simulink model "Filter"  (Simulink 6.5)
settings: Solver=FixedStepDiscrete  StartTime=0.0  StopTime=10.0  RelTol=1e-3
undefined symbols (not defined in the file): dfilt
libraries: dsparch4 x71
(part 1 of 3)
settings Model: Creator=cameraman  LastModifiedBy=cameraman  ExtModeAutoUpdateStatusClock=off
settings OptimizationCC: OptimizeModelRefInitCode=on  LifeSpan=1
settings RTWCC: SystemTargetFile=ert.tlc  TemplateMakefile=ert_default_tmf  Description=Real-Time Workshop Embedded Coder (no auto configuration)  GenerateReport=on  ProcessScript=ert_make_rtw_hook  IncludeHyperlinkInReport=on  LaunchReport=on
settings CodeAppCC: IgnoreCustomStorageClasses=off
settings ERTTargetCC: TargetFcnLib=ansi_tfl_tmw.mat  GenFloatMathFcnCalls=ANSI_C  GenerateSampleERTMain=on  InlinedParameterPlacement=NonHierarchical  ERTCustomFileTemplate=example_file_process.tlc

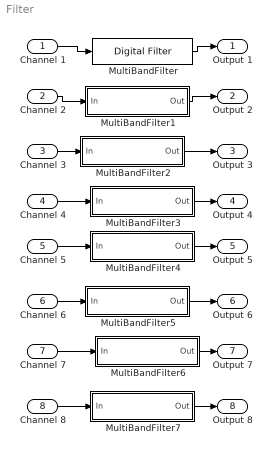
== system Filter ==
  Channel 1 : Inport  PortDimensions=[400 1]  DataType=single
  Channel 2 : Inport  Port=2  PortDimensions=[400 1]  DataType=single
  Channel 3 : Inport  Port=3  PortDimensions=[400 1]  DataType=single
  Channel 4 : Inport  Port=4  PortDimensions=[400 1]  DataType=single
  Channel 5 : Inport  Port=5  PortDimensions=[400 1]  DataType=single
  Channel 6 : Inport  Port=6  PortDimensions=[400 1]  DataType=single
  Channel 7 : Inport  Port=7  PortDimensions=[400 1]  DataType=single
  Channel 8 : Inport  Port=8  PortDimensions=[400 1]  DataType=single
  MultiBandFilter : dsparch4/Digital Filter  Tag=BlockMethodSubSystem  DialogController=dspdialog.DigitalFilter  DialogControllerArgs=DataTag0  TypePopup=IIR (poles & zeros)  IIRFiltStruct=Biquad direct form II (SOS)  AllPoleFiltStruct=Direct form  FIRFiltStruct=Direct form  CoeffSource=Specify via dialog  NumCoeffs=[1 2]  DenCoeffs=[1 0.1]  BiQuadCoeffs=[1 -1.99751859287897 1 1 -1.99114673192373 0.993753760540243;1 -1.99804090685014 0.999999999999999 1 -1.99287686475877 0.994730821052702]  LatticeCoeffs=[0.2 0.4]  denIgnore=on  FiltPerSampPopup=One filter per frame  IC=0  ICnum=0  ICden=0  roundingMode=Floor  overflowMode=off  ScaleValues=[0.994242170508505;1;1]  scaleValueFracLength=14  stageInFracLength=15  stageOutFracLength=15  FilterSource=Specify via dialog  dfiltObjectName=dfilt.dffir([1 2 1])
  MultiBandFilter1 : Subsystem  Tag=BlockMethodSubSystem
  MultiBandFilter2 : Subsystem  Tag=BlockMethodSubSystem
  MultiBandFilter3 : Subsystem  Tag=BlockMethodSubSystem
  MultiBandFilter4 : Subsystem  Tag=BlockMethodSubSystem
  MultiBandFilter5 : Subsystem  Tag=BlockMethodSubSystem
  MultiBandFilter6 : Subsystem  Tag=BlockMethodSubSystem
  MultiBandFilter7 : Subsystem  Tag=BlockMethodSubSystem
  Output 1 : Outport
  Output 2 : Outport  Port=2
  Output 3 : Outport  Port=3
  Output 4 : Outport  Port=4
  Output 5 : Outport  Port=5
  Output 6 : Outport  Port=6
  Output 7 : Outport  Port=7
  Output 8 : Outport  Port=8
  wires:
  Channel 1/1 -> MultiBandFilter/1
  MultiBandFilter/1 -> Output 1/1
  Channel 2/1 -> MultiBandFilter1/1(In)
  MultiBandFilter1/1(Out) -> Output 2/1
  Channel 3/1 -> MultiBandFilter2/1(In)
  MultiBandFilter2/1(Out) -> Output 3/1
  Channel 4/1 -> MultiBandFilter3/1(In)
  MultiBandFilter3/1(Out) -> Output 4/1
  Channel 5/1 -> MultiBandFilter4/1(In)
  MultiBandFilter4/1(Out) -> Output 5/1
  Channel 6/1 -> MultiBandFilter5/1(In)
  MultiBandFilter5/1(Out) -> Output 6/1
  Channel 7/1 -> MultiBandFilter6/1(In)
  MultiBandFilter6/1(Out) -> Output 7/1
  Channel 8/1 -> MultiBandFilter7/1(In)
  MultiBandFilter7/1(Out) -> Output 8/1

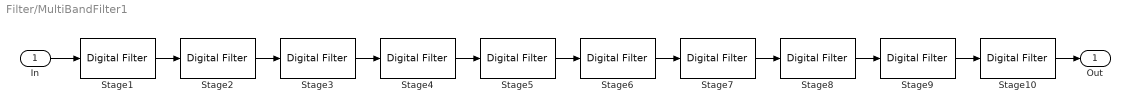
== system Filter/MultiBandFilter1 ==
  In : Inport
  Stage1 : dsparch4/Digital Filter  Tag=BlockMethodSubSystem  DialogController=dspdialog.DigitalFilter  DialogControllerArgs=DataTag1  TypePopup=IIR (poles & zeros)  IIRFiltStruct=Biquad direct form II (SOS)  AllPoleFiltStruct=Direct form  FIRFiltStruct=Direct form  CoeffSource=Specify via dialog  NumCoeffs=[1 2]  DenCoeffs=[1 0.1]  BiQuadCoeffs=[1 -1.99779918117944 1 1 -1.9841893580212 0.986532671822607;1 -1.99779918117944 1 1 -1.9844084470834 0.986594514381433;1 -1.99779918117944 1 1 -1.98482594276861 0.987328003055499;1 -1.99779918117944 1 1 -1.98539047342403 0.987430635535995;1 -1.99779918117944 1 1 -1.98700178992716 0.98891468957857;1 -1.99779918117944 1 1 -1.98634462539793 0.988995338567042;1 -1.99779918117944 1 1 -1.98909486873423 0.990903795973587;1 -1.99779918117944 1 1 -1.98868956515963 0.991466803510252;1 -1.99779918117944 1 1 -1.99152919723188 0.993259885911427;1 -1.99779918117944 1 1 -1.99172030080645 0.994590980134811;1 -1.99779918117944 1 1 -1.99418204154646 0.9958611964492;1 -1.99779918117944 1 1 -1.99522268630609 0.998145251526606;1 -1.99779918117944 1 1 -1.99694953271705 0.998604078200721]  LatticeCoeffs=[0.2 0.4]  denIgnore=on  FiltPerSampPopup=One filter per frame  IC=0  ICnum=0  ICden=0  roundingMode=Floor  overflowMode=off  ScaleValues=[0.94555573617425;1;1;1;1;1;1;1;1;1;1;1;1;1]  scaleValueFracLength=14  stageInFracLength=15  stageOutFracLength=15  FilterSource=Specify via dialog  dfiltObjectName=dfilt.dffir([1 2 1])
  Stage10 : dsparch4/Digital Filter  Tag=BlockMethodSubSystem  DialogController=dspdialog.DigitalFilter  DialogControllerArgs=DataTag2  TypePopup=IIR (poles & zeros)  IIRFiltStruct=Biquad direct form II (SOS)  AllPoleFiltStruct=Direct form  FIRFiltStruct=Direct form  CoeffSource=Specify via dialog  NumCoeffs=[1 2]  DenCoeffs=[1 0.1]  BiQuadCoeffs=[1 -1.78206655900016 1 1 -1.76882371693892 0.986071932968289;1 -1.78206655900016 1 1 -1.77053018639569 0.986121890411467;1 -1.78206655900016 1 1 -1.76800612910907 0.986970023612059;1 -1.78206655900016 1 1 -1.77300273862414 0.987106634145622;1 -1.78206655900016 1 1 -1.76814322166804 0.988766014578574;1 -1.78206655900016 1 1 -1.776071635619 0.98895295803498;1 -1.78206655900016 1 1 -1.7692366984374 0.991346893216688;1 -1.78206655900016 1 1 -1.77953211525407 0.991534308059337;1 -1.78206655900016 1 1 -1.77122117194367 0.994542018120079;1 -1.78206655900016 1 1 -1.78315724552427 0.994679643471267;1 -1.78206655900016 1 1 -1.77396619462103 0.998133320751102;1 -1.78206655900016 1 1 -1.78671109622842 0.998183872576326]  LatticeCoeffs=[0.2 0.4]  denIgnore=on  FiltPerSampPopup=One filter per frame  IC=0  ICnum=0  ICden=0  roundingMode=Floor  overflowMode=off  ScaleValues=[0.947343827190167;1;1;1;1;1;1;1;1;1;1;1;1]  scaleValueFracLength=14  stageInFracLength=15  stageOutFracLength=15  FilterSource=Specify via dialog  dfiltObjectName=dfilt.dffir([1 2 1])
  Stage2 : dsparch4/Digital Filter  Tag=BlockMethodSubSystem  DialogController=dspdialog.DigitalFilter  DialogControllerArgs=DataTag3  TypePopup=IIR (poles & zeros)  IIRFiltStruct=Biquad direct form II (SOS)  AllPoleFiltStruct=Direct form  FIRFiltStruct=Direct form  CoeffSource=Specify via dialog  NumCoeffs=[1 2]  DenCoeffs=[1 0.1]  BiQuadCoeffs=[1 -1.99114895169414 1 1 -1.9777698136482 0.986561389056741;1 -1.99114895169414 1 1 -1.97762596482961 0.986726523617136;1 -1.99114895169414 1 1 -1.97867590148041 0.987172279710376;1 -1.99114895169414 1 1 -1.97829191516836 0.987696909569038;1 -1.99114895169414 1 1 -1.98025580346007 0.98848655327017;1 -1.99114895169414 1 1 -1.97976262159325 0.989447779407759;1 -1.99114895169414 1 1 -1.98239359272873 0.990400910611987;1 -1.99114895169414 1 1 -1.98197315937799 0.99189471261422;1 -1.99114895169414 1 1 -1.98495805169617 0.992793520063566;1 -1.99114895169414 1 1 -1.98479800244236 0.994894776562119;1 -1.99114895169414 1 1 -1.98781178283368 0.995533402367328;1 -1.99114895169414 1 1 -1.98805774118811 0.998255069724644;1 -1.99114895169414 1 1 -1.99081649186752 0.998486141008158]  LatticeCoeffs=[0.2 0.4]  denIgnore=on  FiltPerSampPopup=One filter per frame  IC=0  ICnum=0  ICden=0  roundingMode=Floor  overflowMode=off  ScaleValues=[0.945424059198097;1;1;1;1;1;1;1;1;1;1;1;1;1]  scaleValueFracLength=14  stageInFracLength=15  stageOutFracLength=15  FilterSource=Specify via dialog  dfiltObjectName=dfilt.dffir([1 2 1])
  Stage3 : dsparch4/Digital Filter  Tag=BlockMethodSubSystem  DialogController=dspdialog.DigitalFilter  DialogControllerArgs=DataTag4  TypePopup=IIR (poles & zeros)  IIRFiltStruct=Biquad direct form II (SOS)  AllPoleFiltStruct=Direct form  FIRFiltStruct=Direct form  CoeffSource=Specify via dialog  NumCoeffs=[1 2]  DenCoeffs=[1 0.1]  BiQuadCoeffs=[1 -1.98008133141043 1 1 -1.96672531746014 0.98650963095461;1 -1.98008133141043 1 1 -1.9665032033086 0.986750210536813;1 -1.98008133141043 1 1 -1.96770829457944 0.987048018168876;1 -1.98008133141043 1 1 -1.96708108164623 0.987781888491603;1 -1.98008133141043 1 1 -1.9693722273266 0.988309689218342;1 -1.98008133141043 1 1 -1.96844912868538 0.989566666186125;1 -1.98008133141043 1 1 -1.97160622384232 0.990204155709112;1 -1.98008133141043 1 1 -1.9705438145287 0.992013704878429;1 -1.98008133141043 1 1 -1.97427807467665 0.992615273561397;1 -1.98008133141043 1 1 -1.97324801352515 0.994981712399624;1 -1.98008133141043 1 1 -1.9772425042935 0.995409386053048;1 -1.98008133141043 1 1 -1.97639672748523 0.998286892295906;1 -1.98008133141043 1 1 -1.98034741185451 0.998441686205688]  LatticeCoeffs=[0.2 0.4]  denIgnore=on  FiltPerSampPopup=One filter per frame  IC=0  ICnum=0  ICden=0  roundingMode=Floor  overflowMode=off  ScaleValues=[0.94521834272877;1;1;1;1;1;1;1;1;1;1;1;1;1]  scaleValueFracLength=14  stageInFracLength=15  stageOutFracLength=15  FilterSource=Specify via dialog  dfiltObjectName=dfilt.dffir([1 2 1])
  Stage4 : dsparch4/Digital Filter  Tag=BlockMethodSubSystem  DialogController=dspdialog.DigitalFilter  DialogControllerArgs=DataTag5  TypePopup=IIR (poles & zeros)  IIRFiltStruct=Biquad direct form II (SOS)  AllPoleFiltStruct=Direct form  FIRFiltStruct=Direct form  CoeffSource=Specify via dialog  NumCoeffs=[1 2]  DenCoeffs=[1 0.1]  BiQuadCoeffs=[1 -1.96462073071133 1 1 -1.95131453516727 0.986454183918466;1 -1.96462073071133 1 1 -1.95097599315203 0.986733316047603;1 -1.96462073071133 1 1 -1.95241103954817 0.986957189742735;1 -1.96462073071133 1 1 -1.95143475200162 0.987798186147947;1 -1.96462073071133 1 1 -1.95418555944522 0.988195019819642;1 -1.96462073071133 1 1 -1.95268285779345 0.989604039158267;1 -1.96462073071133 1 1 -1.95652583164486 0.990083454905274;1 -1.96462073071133 1 1 -1.95466134426594 0.992056533195046;1 -1.96462073071133 1 1 -1.95929588143521 0.992509047155787;1 -1.96462073071133 1 1 -1.95726060193215 0.99501482064796;1 -1.96462073071133 1 1 -1.96234396844906 0.995336593760866;1 -1.96462073071133 1 1 -1.96032547879966 0.998299286167002;1 -1.96462073071133 1 1 -1.96550938793341 0.99841576443763]  LatticeCoeffs=[0.2 0.4]  denIgnore=on  FiltPerSampPopup=One filter per frame  IC=0  ICnum=0  ICden=0  roundingMode=Floor  overflowMode=off  ScaleValues=[0.944998002113535;1;1;1;1;1;1;1;1;1;1;1;1;1]  scaleValueFracLength=14  stageInFracLength=15  stageOutFracLength=15  FilterSource=Specify via dialog  dfiltObjectName=dfilt.dffir([1 2 1])
  Stage5 : dsparch4/Digital Filter  Tag=BlockMethodSubSystem  DialogController=dspdialog.DigitalFilter  DialogControllerArgs=DataTag6  TypePopup=IIR (poles & zeros)  IIRFiltStruct=Biquad direct form II (SOS)  AllPoleFiltStruct=Direct form  FIRFiltStruct=Direct form  CoeffSource=Specify via dialog  NumCoeffs=[1 2]  DenCoeffs=[1 0.1]  BiQuadCoeffs=[1 -1.94478249891763 1 1 -1.93168563103253 0.986531277515732;1 -1.94478249891763 1 1 -1.93122059433768 0.98683224264617;1 -1.94478249891763 1 1 -1.93289679174763 0.987008022660797;1 -1.94478249891763 1 1 -1.9315440207779 0.987909159177024;1 -1.94478249891763 1 1 -1.93477174408612 0.988220764886103;1 -1.94478249891763 1 1 -1.93265238090657 0.989713390126836;1 -1.94478249891763 1 1 -1.93719562555007 0.990089878461174;1 -1.94478249891763 1 1 -1.93449307371312 0.99214912798033;1 -1.94478249891763 1 1 -1.94002906949208 0.992504525913789;1 -1.94478249891763 1 1 -1.93696481960067 0.995076908665192;1 -1.94478249891763 1 1 -1.94311601779459 0.995329644404817;1 -1.94478249891763 1 1 -1.93992220998769 0.998321181982756;1 -1.94478249891763 1 1 -1.94629090980952 0.998412672723036]  LatticeCoeffs=[0.2 0.4]  denIgnore=on  FiltPerSampPopup=One filter per frame  IC=0  ICnum=0  ICden=0  roundingMode=Floor  overflowMode=off  ScaleValues=[0.945304374468395;1;1;1;1;1;1;1;1;1;1;1;1;1]  scaleValueFracLength=14  stageInFracLength=15  stageOutFracLength=15  FilterSource=Specify via dialog  dfiltObjectName=dfilt.dffir([1 2 1])
  Stage6 : dsparch4/Digital Filter  Tag=BlockMethodSubSystem  DialogController=dspdialog.DigitalFilter  DialogControllerArgs=DataTag7  TypePopup=IIR (poles & zeros)  IIRFiltStruct=Biquad direct form II (SOS)  AllPoleFiltStruct=Direct form  FIRFiltStruct=Direct form  CoeffSource=Specify via dialog  NumCoeffs=[1 2]  DenCoeffs=[1 0.1]  BiQuadCoeffs=[1 -1.92064508859285 1 1 -1.90765410756011 0.986472273185828;1 -1.92064508859285 1 1 -1.907050442905 0.986789562567385;1 -1.92064508859285 1 1 -1.90899779890478 0.986936076758397;1 -1.92064508859285 1 1 -1.90723446074659 0.987882764412469;1 -1.92064508859285 1 1 -1.91099420923453 0.988142502047033;1 -1.92064508859285 1 1 -1.90820859710794 0.989700395733405;1 -1.92064508859285 1 1 -1.91352351788692 0.990014235945716;1 -1.92064508859285 1 1 -1.90992699967146 0.992144970754847;1 -1.92064508859285 1 1 -1.91644123248104 0.992441250621335;1 -1.92064508859285 1 1 -1.91229576801519 0.995076816055327;1 -1.92064508859285 1 1 -1.91958607166706 0.995287523829068;1 -1.92064508859285 1 1 -1.91517702031526 0.998321590786422;1 -1.92064508859285 1 1 -1.92278752399999 0.998397870496279]  LatticeCoeffs=[0.2 0.4]  denIgnore=on  FiltPerSampPopup=One filter per frame  IC=0  ICnum=0  ICden=0  roundingMode=Floor  overflowMode=off  ScaleValues=[0.94506988263773;1;1;1;1;1;1;1;1;1;1;1;1;1]  scaleValueFracLength=14  stageInFracLength=15  stageOutFracLength=15  FilterSource=Specify via dialog  dfiltObjectName=dfilt.dffir([1 2 1])
  Stage7 : dsparch4/Digital Filter  Tag=BlockMethodSubSystem  DialogController=dspdialog.DigitalFilter  DialogControllerArgs=DataTag8  TypePopup=IIR (poles & zeros)  IIRFiltStruct=Biquad direct form II (SOS)  AllPoleFiltStruct=Direct form  FIRFiltStruct=Direct form  CoeffSource=Specify via dialog  NumCoeffs=[1 2]  DenCoeffs=[1 0.1]  BiQuadCoeffs=[1 -1.89222757165677 1 1 -1.87946492530582 0.986510453032056;1 -1.89222757165677 1 1 -1.87872413047093 0.986838101460465;1 -1.89222757165677 1 1 -1.88093278114135 0.986961705641337;1 -1.89222757165677 1 1 -1.87876382191273 0.987936924736541;1 -1.89222757165677 1 1 -1.88303530627035 0.988156052672692;1 -1.89222757165677 1 1 -1.87959304768991 0.989753596101735;1 -1.89222757165677 1 1 -1.88564809933575 0.990018375641976;1 -1.89222757165677 1 1 -1.88117342448449 0.992189935251698;1 -1.89222757165677 1 1 -1.88862249944903 0.992439907123505;1 -1.89222757165677 1 1 -1.88341916121208 0.995106934972423;1 -1.89222757165677 1 1 -1.89179355317212 0.99528471353657;1 -1.89222757165677 1 1 -1.88620064251826 0.998332207367685;1 -1.89222757165677 1 1 -1.89498786374351 0.998396566697007]  LatticeCoeffs=[0.2 0.4]  denIgnore=on  FiltPerSampPopup=One filter per frame  IC=0  ICnum=0  ICden=0  roundingMode=Floor  overflowMode=off  ScaleValues=[0.945221609871693;1;1;1;1;1;1;1;1;1;1;1;1;1]  scaleValueFracLength=14  stageInFracLength=15  stageOutFracLength=15  FilterSource=Specify via dialog  dfiltObjectName=dfilt.dffir([1 2 1])
  Stage8 : dsparch4/Digital Filter  Tag=BlockMethodSubSystem  DialogController=dspdialog.DigitalFilter  DialogControllerArgs=DataTag9  TypePopup=IIR (poles & zeros)  IIRFiltStruct=Biquad direct form II (SOS)  AllPoleFiltStruct=Direct form  FIRFiltStruct=Direct form  CoeffSource=Specify via dialog  NumCoeffs=[1 2]  DenCoeffs=[1 0.1]  BiQuadCoeffs=[1 -1.85960883542276 1 1 -1.84593411646957 0.986021509148453;1 -1.85960883542276 1 1 -1.84734605082752 0.986086207824345;1 -1.85960883542276 1 1 -1.84544140778377 0.986909714475135;1 -1.85960883542276 1 1 -1.84957097535378 0.987086633043367;1 -1.85960883542276 1 1 -1.84591485590852 0.9887038952601;1 -1.85960883542276 1 1 -1.85245319647007 0.988945992272582;1 -1.85960883542276 1 1 -1.8473354240394 0.991292677324705;1 -1.85960883542276 1 1 -1.85579926237776 0.991535378665241;1 -1.85960883542276 1 1 -1.84961594661188 0.994504963105796;1 -1.85960883542276 1 1 -1.85939042619789 0.994683183912115;1 -1.85960883542276 1 1 -1.85260449337881 0.998120129074157;1 -1.85960883542276 1 1 -1.86299517573272 0.998185591844758]  LatticeCoeffs=[0.2 0.4]  denIgnore=on  FiltPerSampPopup=One filter per frame  IC=0  ICnum=0  ICden=0  roundingMode=Floor  overflowMode=off  ScaleValues=[0.947184039013874;1;1;1;1;1;1;1;1;1;1;1;1]  scaleValueFracLength=14  stageInFracLength=15  stageOutFracLength=15  FilterSource=Specify via dialog  dfiltObjectName=dfilt.dffir([1 2 1])
  Stage9 : dsparch4/Digital Filter  Tag=BlockMethodSubSystem  DialogController=dspdialog.DigitalFilter  DialogControllerArgs=DataTag10  TypePopup=IIR (poles & zeros)  IIRFiltStruct=Biquad direct form II (SOS)  AllPoleFiltStruct=Direct form  FIRFiltStruct=Direct form  CoeffSource=Specify via dialog  NumCoeffs=[1 2]  DenCoeffs=[1 0.1]  BiQuadCoeffs=[1 -1.82286130163383 1 1 -1.8093904390343 0.986049340185928;1 -1.82286130163383 1 1 -1.81095051165661 0.986105875757923;1 -1.82286130163383 1 1 -1.80873514996766 0.986943025633069;1 -1.82286130163383 1 1 -1.81330095324135 0.987097623443224;1 -1.82286130163383 1 1 -1.80904088159003 0.988738220453347;1 -1.82286130163383 1 1 -1.81627907594021 0.988949776437469;1 -1.82286130163383 1 1 -1.81029885913928 0.991322642616634;1 -1.82286130163383 1 1 -1.81968568641089 0.991534729877009;1 -1.82286130163383 1 1 -1.81243274513281 0.994525446348993;1 -1.82286130163383 1 1 -1.82329772701486 0.994681188352925;1 -1.82286130163383 1 1 -1.8153013406224 0.998127421634027;1 -1.82286130163383 1 1 -1.82688113842232 0.998184627861444]  LatticeCoeffs=[0.2 0.4]  denIgnore=on  FiltPerSampPopup=One filter per frame  IC=0  ICnum=0  ICden=0  roundingMode=Floor  overflowMode=off  ScaleValues=[0.947272180688283;1;1;1;1;1;1;1;1;1;1;1;1]  scaleValueFracLength=14  stageInFracLength=15  stageOutFracLength=15  FilterSource=Specify via dialog  dfiltObjectName=dfilt.dffir([1 2 1])
  Out : Outport
  wires:
  In/1 -> Stage1/1
  Stage1/1 -> Stage2/1
  Stage2/1 -> Stage3/1
  Stage3/1 -> Stage4/1
  Stage4/1 -> Stage5/1
  Stage5/1 -> Stage6/1
  Stage6/1 -> Stage7/1
  Stage7/1 -> Stage8/1
  Stage8/1 -> Stage9/1
  Stage9/1 -> Stage10/1
  Stage10/1 -> Out/1

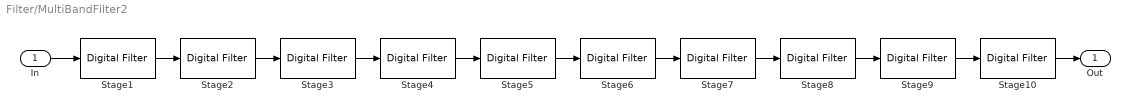
== system Filter/MultiBandFilter2 ==
  In : Inport
  Stage1 : dsparch4/Digital Filter  Tag=BlockMethodSubSystem  DialogController=dspdialog.DigitalFilter  DialogControllerArgs=DataTag11  TypePopup=IIR (poles & zeros)  IIRFiltStruct=Biquad direct form II (SOS)  AllPoleFiltStruct=Direct form  FIRFiltStruct=Direct form  CoeffSource=Specify via dialog  NumCoeffs=[1 2]  DenCoeffs=[1 0.1]  BiQuadCoeffs=[1 -1.99779918117944 1 1 -1.9841893580212 0.986532671822607;1 -1.99779918117944 1 1 -1.9844084470834 0.986594514381433;1 -1.99779918117944 1 1 -1.98482594276861 0.987328003055499;1 -1.99779918117944 1 1 -1.98539047342403 0.987430635535995;1 -1.99779918117944 1 1 -1.98700178992716 0.98891468957857;1 -1.99779918117944 1 1 -1.98634462539793 0.988995338567042;1 -1.99779918117944 1 1 -1.98909486873423 0.990903795973587;1 -1.99779918117944 1 1 -1.98868956515963 0.991466803510252;1 -1.99779918117944 1 1 -1.99152919723188 0.993259885911427;1 -1.99779918117944 1 1 -1.99172030080645 0.994590980134811;1 -1.99779918117944 1 1 -1.99418204154646 0.9958611964492;1 -1.99779918117944 1 1 -1.99522268630609 0.998145251526606;1 -1.99779918117944 1 1 -1.99694953271705 0.998604078200721]  LatticeCoeffs=[0.2 0.4]  denIgnore=on  FiltPerSampPopup=One filter per frame  IC=0  ICnum=0  ICden=0  roundingMode=Floor  overflowMode=off  ScaleValues=[0.94555573617425;1;1;1;1;1;1;1;1;1;1;1;1;1]  scaleValueFracLength=14  stageInFracLength=15  stageOutFracLength=15  FilterSource=Specify via dialog  dfiltObjectName=dfilt.dffir([1 2 1])
  Stage10 : dsparch4/Digital Filter  Tag=BlockMethodSubSystem  DialogController=dspdialog.DigitalFilter  DialogControllerArgs=DataTag12  TypePopup=IIR (poles & zeros)  IIRFiltStruct=Biquad direct form II (SOS)  AllPoleFiltStruct=Direct form  FIRFiltStruct=Direct form  CoeffSource=Specify via dialog  NumCoeffs=[1 2]  DenCoeffs=[1 0.1]  BiQuadCoeffs=[1 -1.78206655900016 1 1 -1.76882371693892 0.986071932968289;1 -1.78206655900016 1 1 -1.77053018639569 0.986121890411467;1 -1.78206655900016 1 1 -1.76800612910907 0.986970023612059;1 -1.78206655900016 1 1 -1.77300273862414 0.987106634145622;1 -1.78206655900016 1 1 -1.76814322166804 0.988766014578574;1 -1.78206655900016 1 1 -1.776071635619 0.98895295803498;1 -1.78206655900016 1 1 -1.7692366984374 0.991346893216688;1 -1.78206655900016 1 1 -1.77953211525407 0.991534308059337;1 -1.78206655900016 1 1 -1.77122117194367 0.994542018120079;1 -1.78206655900016 1 1 -1.78315724552427 0.994679643471267;1 -1.78206655900016 1 1 -1.77396619462103 0.998133320751102;1 -1.78206655900016 1 1 -1.78671109622842 0.998183872576326]  LatticeCoeffs=[0.2 0.4]  denIgnore=on  FiltPerSampPopup=One filter per frame  IC=0  ICnum=0  ICden=0  roundingMode=Floor  overflowMode=off  ScaleValues=[0.947343827190167;1;1;1;1;1;1;1;1;1;1;1;1]  scaleValueFracLength=14  stageInFracLength=15  stageOutFracLength=15  FilterSource=Specify via dialog  dfiltObjectName=dfilt.dffir([1 2 1])
  Stage2 : dsparch4/Digital Filter  Tag=BlockMethodSubSystem  DialogController=dspdialog.DigitalFilter  DialogControllerArgs=DataTag13  TypePopup=IIR (poles & zeros)  IIRFiltStruct=Biquad direct form II (SOS)  AllPoleFiltStruct=Direct form  FIRFiltStruct=Direct form  CoeffSource=Specify via dialog  NumCoeffs=[1 2]  DenCoeffs=[1 0.1]  BiQuadCoeffs=[1 -1.99114895169414 1 1 -1.9777698136482 0.986561389056741;1 -1.99114895169414 1 1 -1.97762596482961 0.986726523617136;1 -1.99114895169414 1 1 -1.97867590148041 0.987172279710376;1 -1.99114895169414 1 1 -1.97829191516836 0.987696909569038;1 -1.99114895169414 1 1 -1.98025580346007 0.98848655327017;1 -1.99114895169414 1 1 -1.97976262159325 0.989447779407759;1 -1.99114895169414 1 1 -1.98239359272873 0.990400910611987;1 -1.99114895169414 1 1 -1.98197315937799 0.99189471261422;1 -1.99114895169414 1 1 -1.98495805169617 0.992793520063566;1 -1.99114895169414 1 1 -1.98479800244236 0.994894776562119;1 -1.99114895169414 1 1 -1.98781178283368 0.995533402367328;1 -1.99114895169414 1 1 -1.98805774118811 0.998255069724644;1 -1.99114895169414 1 1 -1.99081649186752 0.998486141008158]  LatticeCoeffs=[0.2 0.4]  denIgnore=on  FiltPerSampPopup=One filter per frame  IC=0  ICnum=0  ICden=0  roundingMode=Floor  overflowMode=off  ScaleValues=[0.945424059198097;1;1;1;1;1;1;1;1;1;1;1;1;1]  scaleValueFracLength=14  stageInFracLength=15  stageOutFracLength=15  FilterSource=Specify via dialog  dfiltObjectName=dfilt.dffir([1 2 1])
  Stage3 : dsparch4/Digital Filter  Tag=BlockMethodSubSystem  DialogController=dspdialog.DigitalFilter  DialogControllerArgs=DataTag14  TypePopup=IIR (poles & zeros)  IIRFiltStruct=Biquad direct form II (SOS)  AllPoleFiltStruct=Direct form  FIRFiltStruct=Direct form  CoeffSource=Specify via dialog  NumCoeffs=[1 2]  DenCoeffs=[1 0.1]  BiQuadCoeffs=[1 -1.98008133141043 1 1 -1.96672531746014 0.98650963095461;1 -1.98008133141043 1 1 -1.9665032033086 0.986750210536813;1 -1.98008133141043 1 1 -1.96770829457944 0.987048018168876;1 -1.98008133141043 1 1 -1.96708108164623 0.987781888491603;1 -1.98008133141043 1 1 -1.9693722273266 0.988309689218342;1 -1.98008133141043 1 1 -1.96844912868538 0.989566666186125;1 -1.98008133141043 1 1 -1.97160622384232 0.990204155709112;1 -1.98008133141043 1 1 -1.9705438145287 0.992013704878429;1 -1.98008133141043 1 1 -1.97427807467665 0.992615273561397;1 -1.98008133141043 1 1 -1.97324801352515 0.994981712399624;1 -1.98008133141043 1 1 -1.9772425042935 0.995409386053048;1 -1.98008133141043 1 1 -1.97639672748523 0.998286892295906;1 -1.98008133141043 1 1 -1.98034741185451 0.998441686205688]  LatticeCoeffs=[0.2 0.4]  denIgnore=on  FiltPerSampPopup=One filter per frame  IC=0  ICnum=0  ICden=0  roundingMode=Floor  overflowMode=off  ScaleValues=[0.94521834272877;1;1;1;1;1;1;1;1;1;1;1;1;1]  scaleValueFracLength=14  stageInFracLength=15  stageOutFracLength=15  FilterSource=Specify via dialog  dfiltObjectName=dfilt.dffir([1 2 1])
  Stage4 : dsparch4/Digital Filter  Tag=BlockMethodSubSystem  DialogController=dspdialog.DigitalFilter  DialogControllerArgs=DataTag15  TypePopup=IIR (poles & zeros)  IIRFiltStruct=Biquad direct form II (SOS)  AllPoleFiltStruct=Direct form  FIRFiltStruct=Direct form  CoeffSource=Specify via dialog  NumCoeffs=[1 2]  DenCoeffs=[1 0.1]  BiQuadCoeffs=[1 -1.96462073071133 1 1 -1.95131453516727 0.986454183918466;1 -1.96462073071133 1 1 -1.95097599315203 0.986733316047603;1 -1.96462073071133 1 1 -1.95241103954817 0.986957189742735;1 -1.96462073071133 1 1 -1.95143475200162 0.987798186147947;1 -1.96462073071133 1 1 -1.95418555944522 0.988195019819642;1 -1.96462073071133 1 1 -1.95268285779345 0.989604039158267;1 -1.96462073071133 1 1 -1.95652583164486 0.990083454905274;1 -1.96462073071133 1 1 -1.95466134426594 0.992056533195046;1 -1.96462073071133 1 1 -1.95929588143521 0.992509047155787;1 -1.96462073071133 1 1 -1.95726060193215 0.99501482064796;1 -1.96462073071133 1 1 -1.96234396844906 0.995336593760866;1 -1.96462073071133 1 1 -1.96032547879966 0.998299286167002;1 -1.96462073071133 1 1 -1.96550938793341 0.99841576443763]  LatticeCoeffs=[0.2 0.4]  denIgnore=on  FiltPerSampPopup=One filter per frame  IC=0  ICnum=0  ICden=0  roundingMode=Floor  overflowMode=off  ScaleValues=[0.944998002113535;1;1;1;1;1;1;1;1;1;1;1;1;1]  scaleValueFracLength=14  stageInFracLength=15  stageOutFracLength=15  FilterSource=Specify via dialog  dfiltObjectName=dfilt.dffir([1 2 1])
  Stage5 : dsparch4/Digital Filter  Tag=BlockMethodSubSystem  DialogController=dspdialog.DigitalFilter  DialogControllerArgs=DataTag16  TypePopup=IIR (poles & zeros)  IIRFiltStruct=Biquad direct form II (SOS)  AllPoleFiltStruct=Direct form  FIRFiltStruct=Direct form  CoeffSource=Specify via dialog  NumCoeffs=[1 2]  DenCoeffs=[1 0.1]  BiQuadCoeffs=[1 -1.94478249891763 1 1 -1.93168563103253 0.986531277515732;1 -1.94478249891763 1 1 -1.93122059433768 0.98683224264617;1 -1.94478249891763 1 1 -1.93289679174763 0.987008022660797;1 -1.94478249891763 1 1 -1.9315440207779 0.987909159177024;1 -1.94478249891763 1 1 -1.93477174408612 0.988220764886103;1 -1.94478249891763 1 1 -1.93265238090657 0.989713390126836;1 -1.94478249891763 1 1 -1.93719562555007 0.990089878461174;1 -1.94478249891763 1 1 -1.93449307371312 0.99214912798033;1 -1.94478249891763 1 1 -1.94002906949208 0.992504525913789;1 -1.94478249891763 1 1 -1.93696481960067 0.995076908665192;1 -1.94478249891763 1 1 -1.94311601779459 0.995329644404817;1 -1.94478249891763 1 1 -1.93992220998769 0.998321181982756;1 -1.94478249891763 1 1 -1.94629090980952 0.998412672723036]  LatticeCoeffs=[0.2 0.4]  denIgnore=on  FiltPerSampPopup=One filter per frame  IC=0  ICnum=0  ICden=0  roundingMode=Floor  overflowMode=off  ScaleValues=[0.945304374468395;1;1;1;1;1;1;1;1;1;1;1;1;1]  scaleValueFracLength=14  stageInFracLength=15  stageOutFracLength=15  FilterSource=Specify via dialog  dfiltObjectName=dfilt.dffir([1 2 1])
  Stage6 : dsparch4/Digital Filter  Tag=BlockMethodSubSystem  DialogController=dspdialog.DigitalFilter  DialogControllerArgs=DataTag17  TypePopup=IIR (poles & zeros)  IIRFiltStruct=Biquad direct form II (SOS)  AllPoleFiltStruct=Direct form  FIRFiltStruct=Direct form  CoeffSource=Specify via dialog  NumCoeffs=[1 2]  DenCoeffs=[1 0.1]  BiQuadCoeffs=[1 -1.92064508859285 1 1 -1.90765410756011 0.986472273185828;1 -1.92064508859285 1 1 -1.907050442905 0.986789562567385;1 -1.92064508859285 1 1 -1.90899779890478 0.986936076758397;1 -1.92064508859285 1 1 -1.90723446074659 0.987882764412469;1 -1.92064508859285 1 1 -1.91099420923453 0.988142502047033;1 -1.92064508859285 1 1 -1.90820859710794 0.989700395733405;1 -1.92064508859285 1 1 -1.91352351788692 0.990014235945716;1 -1.92064508859285 1 1 -1.90992699967146 0.992144970754847;1 -1.92064508859285 1 1 -1.91644123248104 0.992441250621335;1 -1.92064508859285 1 1 -1.91229576801519 0.995076816055327;1 -1.92064508859285 1 1 -1.91958607166706 0.995287523829068;1 -1.92064508859285 1 1 -1.91517702031526 0.998321590786422;1 -1.92064508859285 1 1 -1.92278752399999 0.998397870496279]  LatticeCoeffs=[0.2 0.4]  denIgnore=on  FiltPerSampPopup=One filter per frame  IC=0  ICnum=0  ICden=0  roundingMode=Floor  overflowMode=off  ScaleValues=[0.94506988263773;1;1;1;1;1;1;1;1;1;1;1;1;1]  scaleValueFracLength=14  stageInFracLength=15  stageOutFracLength=15  FilterSource=Specify via dialog  dfiltObjectName=dfilt.dffir([1 2 1])
  Stage7 : dsparch4/Digital Filter  Tag=BlockMethodSubSystem  DialogController=dspdialog.DigitalFilter  DialogControllerArgs=DataTag18  TypePopup=IIR (poles & zeros)  IIRFiltStruct=Biquad direct form II (SOS)  AllPoleFiltStruct=Direct form  FIRFiltStruct=Direct form  CoeffSource=Specify via dialog  NumCoeffs=[1 2]  DenCoeffs=[1 0.1]  BiQuadCoeffs=[1 -1.89222757165677 1 1 -1.87946492530582 0.986510453032056;1 -1.89222757165677 1 1 -1.87872413047093 0.986838101460465;1 -1.89222757165677 1 1 -1.88093278114135 0.986961705641337;1 -1.89222757165677 1 1 -1.87876382191273 0.987936924736541;1 -1.89222757165677 1 1 -1.88303530627035 0.988156052672692;1 -1.89222757165677 1 1 -1.87959304768991 0.989753596101735;1 -1.89222757165677 1 1 -1.88564809933575 0.990018375641976;1 -1.89222757165677 1 1 -1.88117342448449 0.992189935251698;1 -1.89222757165677 1 1 -1.88862249944903 0.992439907123505;1 -1.89222757165677 1 1 -1.88341916121208 0.995106934972423;1 -1.89222757165677 1 1 -1.89179355317212 0.99528471353657;1 -1.89222757165677 1 1 -1.88620064251826 0.998332207367685;1 -1.89222757165677 1 1 -1.89498786374351 0.998396566697007]  LatticeCoeffs=[0.2 0.4]  denIgnore=on  FiltPerSampPopup=One filter per frame  IC=0  ICnum=0  ICden=0  roundingMode=Floor  overflowMode=off  ScaleValues=[0.945221609871693;1;1;1;1;1;1;1;1;1;1;1;1;1]  scaleValueFracLength=14  stageInFracLength=15  stageOutFracLength=15  FilterSource=Specify via dialog  dfiltObjectName=dfilt.dffir([1 2 1])
  Stage8 : dsparch4/Digital Filter  Tag=BlockMethodSubSystem  DialogController=dspdialog.DigitalFilter  DialogControllerArgs=DataTag19  TypePopup=IIR (poles & zeros)  IIRFiltStruct=Biquad direct form II (SOS)  AllPoleFiltStruct=Direct form  FIRFiltStruct=Direct form  CoeffSource=Specify via dialog  NumCoeffs=[1 2]  DenCoeffs=[1 0.1]  BiQuadCoeffs=[1 -1.85960883542276 1 1 -1.84593411646957 0.986021509148453;1 -1.85960883542276 1 1 -1.84734605082752 0.986086207824345;1 -1.85960883542276 1 1 -1.84544140778377 0.986909714475135;1 -1.85960883542276 1 1 -1.84957097535378 0.987086633043367;1 -1.85960883542276 1 1 -1.84591485590852 0.9887038952601;1 -1.85960883542276 1 1 -1.85245319647007 0.988945992272582;1 -1.85960883542276 1 1 -1.8473354240394 0.991292677324705;1 -1.85960883542276 1 1 -1.85579926237776 0.991535378665241;1 -1.85960883542276 1 1 -1.84961594661188 0.994504963105796;1 -1.85960883542276 1 1 -1.85939042619789 0.994683183912115;1 -1.85960883542276 1 1 -1.85260449337881 0.998120129074157;1 -1.85960883542276 1 1 -1.86299517573272 0.998185591844758]  LatticeCoeffs=[0.2 0.4]  denIgnore=on  FiltPerSampPopup=One filter per frame  IC=0  ICnum=0  ICden=0  roundingMode=Floor  overflowMode=off  ScaleValues=[0.947184039013874;1;1;1;1;1;1;1;1;1;1;1;1]  scaleValueFracLength=14  stageInFracLength=15  stageOutFracLength=15  FilterSource=Specify via dialog  dfiltObjectName=dfilt.dffir([1 2 1])
  Stage9 : dsparch4/Digital Filter  Tag=BlockMethodSubSystem  DialogController=dspdialog.DigitalFilter  DialogControllerArgs=DataTag20  TypePopup=IIR (poles & zeros)  IIRFiltStruct=Biquad direct form II (SOS)  AllPoleFiltStruct=Direct form  FIRFiltStruct=Direct form  CoeffSource=Specify via dialog  NumCoeffs=[1 2]  DenCoeffs=[1 0.1]  BiQuadCoeffs=[1 -1.82286130163383 1 1 -1.8093904390343 0.986049340185928;1 -1.82286130163383 1 1 -1.81095051165661 0.986105875757923;1 -1.82286130163383 1 1 -1.80873514996766 0.986943025633069;1 -1.82286130163383 1 1 -1.81330095324135 0.987097623443224;1 -1.82286130163383 1 1 -1.80904088159003 0.988738220453347;1 -1.82286130163383 1 1 -1.81627907594021 0.988949776437469;1 -1.82286130163383 1 1 -1.81029885913928 0.991322642616634;1 -1.82286130163383 1 1 -1.81968568641089 0.991534729877009;1 -1.82286130163383 1 1 -1.81243274513281 0.994525446348993;1 -1.82286130163383 1 1 -1.82329772701486 0.994681188352925;1 -1.82286130163383 1 1 -1.8153013406224 0.998127421634027;1 -1.82286130163383 1 1 -1.82688113842232 0.998184627861444]  LatticeCoeffs=[0.2 0.4]  denIgnore=on  FiltPerSampPopup=One filter per frame  IC=0  ICnum=0  ICden=0  roundingMode=Floor  overflowMode=off  ScaleValues=[0.947272180688283;1;1;1;1;1;1;1;1;1;1;1;1]  scaleValueFracLength=14  stageInFracLength=15  stageOutFracLength=15  FilterSource=Specify via dialog  dfiltObjectName=dfilt.dffir([1 2 1])
  Out : Outport
  wires:
  In/1 -> Stage1/1
  Stage1/1 -> Stage2/1
  Stage2/1 -> Stage3/1
  Stage3/1 -> Stage4/1
  Stage4/1 -> Stage5/1
  Stage5/1 -> Stage6/1
  Stage6/1 -> Stage7/1
  Stage7/1 -> Stage8/1
  Stage8/1 -> Stage9/1
  Stage9/1 -> Stage10/1
  Stage10/1 -> Out/1

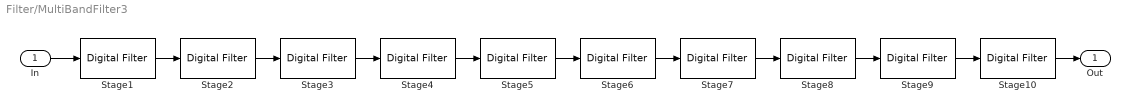
== system Filter/MultiBandFilter3 ==
  In : Inport
  Stage1 : dsparch4/Digital Filter  Tag=BlockMethodSubSystem  DialogController=dspdialog.DigitalFilter  DialogControllerArgs=DataTag21  TypePopup=IIR (poles & zeros)  IIRFiltStruct=Biquad direct form II (SOS)  AllPoleFiltStruct=Direct form  FIRFiltStruct=Direct form  CoeffSource=Specify via dialog  NumCoeffs=[1 2]  DenCoeffs=[1 0.1]  BiQuadCoeffs=[1 -1.99779918117944 1 1 -1.9841893580212 0.986532671822607;1 -1.99779918117944 1 1 -1.9844084470834 0.986594514381433;1 -1.99779918117944 1 1 -1.98482594276861 0.987328003055499;1 -1.99779918117944 1 1 -1.98539047342403 0.987430635535995;1 -1.99779918117944 1 1 -1.98700178992716 0.98891468957857;1 -1.99779918117944 1 1 -1.98634462539793 0.988995338567042;1 -1.99779918117944 1 1 -1.98909486873423 0.990903795973587;1 -1.99779918117944 1 1 -1.98868956515963 0.991466803510252;1 -1.99779918117944 1 1 -1.99152919723188 0.993259885911427;1 -1.99779918117944 1 1 -1.99172030080645 0.994590980134811;1 -1.99779918117944 1 1 -1.99418204154646 0.9958611964492;1 -1.99779918117944 1 1 -1.99522268630609 0.998145251526606;1 -1.99779918117944 1 1 -1.99694953271705 0.998604078200721]  LatticeCoeffs=[0.2 0.4]  denIgnore=on  FiltPerSampPopup=One filter per frame  IC=0  ICnum=0  ICden=0  roundingMode=Floor  overflowMode=off  ScaleValues=[0.94555573617425;1;1;1;1;1;1;1;1;1;1;1;1;1]  scaleValueFracLength=14  stageInFracLength=15  stageOutFracLength=15  FilterSource=Specify via dialog  dfiltObjectName=dfilt.dffir([1 2 1])
  Stage10 : dsparch4/Digital Filter  Tag=BlockMethodSubSystem  DialogController=dspdialog.DigitalFilter  DialogControllerArgs=DataTag22  TypePopup=IIR (poles & zeros)  IIRFiltStruct=Biquad direct form II (SOS)  AllPoleFiltStruct=Direct form  FIRFiltStruct=Direct form  CoeffSource=Specify via dialog  NumCoeffs=[1 2]  DenCoeffs=[1 0.1]  BiQuadCoeffs=[1 -1.78206655900016 1 1 -1.76882371693892 0.986071932968289;1 -1.78206655900016 1 1 -1.77053018639569 0.986121890411467;1 -1.78206655900016 1 1 -1.76800612910907 0.986970023612059;1 -1.78206655900016 1 1 -1.77300273862414 0.987106634145622;1 -1.78206655900016 1 1 -1.76814322166804 0.988766014578574;1 -1.78206655900016 1 1 -1.776071635619 0.98895295803498;1 -1.78206655900016 1 1 -1.7692366984374 0.991346893216688;1 -1.78206655900016 1 1 -1.77953211525407 0.991534308059337;1 -1.78206655900016 1 1 -1.77122117194367 0.994542018120079;1 -1.78206655900016 1 1 -1.78315724552427 0.994679643471267;1 -1.78206655900016 1 1 -1.77396619462103 0.998133320751102;1 -1.78206655900016 1 1 -1.78671109622842 0.998183872576326]  LatticeCoeffs=[0.2 0.4]  denIgnore=on  FiltPerSampPopup=One filter per frame  IC=0  ICnum=0  ICden=0  roundingMode=Floor  overflowMode=off  ScaleValues=[0.947343827190167;1;1;1;1;1;1;1;1;1;1;1;1]  scaleValueFracLength=14  stageInFracLength=15  stageOutFracLength=15  FilterSource=Specify via dialog  dfiltObjectName=dfilt.dffir([1 2 1])
  Stage2 : dsparch4/Digital Filter  Tag=BlockMethodSubSystem  DialogController=dspdialog.DigitalFilter  DialogControllerArgs=DataTag23  TypePopup=IIR (poles & zeros)  IIRFiltStruct=Biquad direct form II (SOS)  AllPoleFiltStruct=Direct form  FIRFiltStruct=Direct form  CoeffSource=Specify via dialog  NumCoeffs=[1 2]  DenCoeffs=[1 0.1]  BiQuadCoeffs=[1 -1.99114895169414 1 1 -1.9777698136482 0.986561389056741;1 -1.99114895169414 1 1 -1.97762596482961 0.986726523617136;1 -1.99114895169414 1 1 -1.97867590148041 0.987172279710376;1 -1.99114895169414 1 1 -1.97829191516836 0.987696909569038;1 -1.99114895169414 1 1 -1.98025580346007 0.98848655327017;1 -1.99114895169414 1 1 -1.97976262159325 0.989447779407759;1 -1.99114895169414 1 1 -1.98239359272873 0.990400910611987;1 -1.99114895169414 1 1 -1.98197315937799 0.99189471261422;1 -1.99114895169414 1 1 -1.98495805169617 0.992793520063566;1 -1.99114895169414 1 1 -1.98479800244236 0.994894776562119;1 -1.99114895169414 1 1 -1.98781178283368 0.995533402367328;1 -1.99114895169414 1 1 -1.98805774118811 0.998255069724644;1 -1.99114895169414 1 1 -1.99081649186752 0.998486141008158]  LatticeCoeffs=[0.2 0.4]  denIgnore=on  FiltPerSampPopup=One filter per frame  IC=0  ICnum=0  ICden=0  roundingMode=Floor  overflowMode=off  ScaleValues=[0.945424059198097;1;1;1;1;1;1;1;1;1;1;1;1;1]  scaleValueFracLength=14  stageInFracLength=15  stageOutFracLength=15  FilterSource=Specify via dialog  dfiltObjectName=dfilt.dffir([1 2 1])
  Stage3 : dsparch4/Digital Filter  Tag=BlockMethodSubSystem  DialogController=dspdialog.DigitalFilter  DialogControllerArgs=DataTag24  TypePopup=IIR (poles & zeros)  IIRFiltStruct=Biquad direct form II (SOS)  AllPoleFiltStruct=Direct form  FIRFiltStruct=Direct form  CoeffSource=Specify via dialog  NumCoeffs=[1 2]  DenCoeffs=[1 0.1]  BiQuadCoeffs=[1 -1.98008133141043 1 1 -1.96672531746014 0.98650963095461;1 -1.98008133141043 1 1 -1.9665032033086 0.986750210536813;1 -1.98008133141043 1 1 -1.96770829457944 0.987048018168876;1 -1.98008133141043 1 1 -1.96708108164623 0.987781888491603;1 -1.98008133141043 1 1 -1.9693722273266 0.988309689218342;1 -1.98008133141043 1 1 -1.96844912868538 0.989566666186125;1 -1.98008133141043 1 1 -1.97160622384232 0.990204155709112;1 -1.98008133141043 1 1 -1.9705438145287 0.992013704878429;1 -1.98008133141043 1 1 -1.97427807467665 0.992615273561397;1 -1.98008133141043 1 1 -1.97324801352515 0.994981712399624;1 -1.98008133141043 1 1 -1.9772425042935 0.995409386053048;1 -1.98008133141043 1 1 -1.97639672748523 0.998286892295906;1 -1.98008133141043 1 1 -1.98034741185451 0.998441686205688]  LatticeCoeffs=[0.2 0.4]  denIgnore=on  FiltPerSampPopup=One filter per frame  IC=0  ICnum=0  ICden=0  roundingMode=Floor  overflowMode=off  ScaleValues=[0.94521834272877;1;1;1;1;1;1;1;1;1;1;1;1;1]  scaleValueFracLength=14  stageInFracLength=15  stageOutFracLength=15  FilterSource=Specify via dialog  dfiltObjectName=dfilt.dffir([1 2 1])
  Stage4 : dsparch4/Digital Filter  Tag=BlockMethodSubSystem  DialogController=dspdialog.DigitalFilter  DialogControllerArgs=DataTag25  TypePopup=IIR (poles & zeros)  IIRFiltStruct=Biquad direct form II (SOS)  AllPoleFiltStruct=Direct form  FIRFiltStruct=Direct form  CoeffSource=Specify via dialog  NumCoeffs=[1 2]  DenCoeffs=[1 0.1]  BiQuadCoeffs=[1 -1.96462073071133 1 1 -1.95131453516727 0.986454183918466;1 -1.96462073071133 1 1 -1.95097599315203 0.986733316047603;1 -1.96462073071133 1 1 -1.95241103954817 0.986957189742735;1 -1.96462073071133 1 1 -1.95143475200162 0.987798186147947;1 -1.96462073071133 1 1 -1.95418555944522 0.988195019819642;1 -1.96462073071133 1 1 -1.95268285779345 0.989604039158267;1 -1.96462073071133 1 1 -1.95652583164486 0.990083454905274;1 -1.96462073071133 1 1 -1.95466134426594 0.992056533195046;1 -1.96462073071133 1 1 -1.95929588143521 0.992509047155787;1 -1.96462073071133 1 1 -1.95726060193215 0.99501482064796;1 -1.96462073071133 1 1 -1.96234396844906 0.995336593760866;1 -1.96462073071133 1 1 -1.96032547879966 0.998299286167002;1 -1.96462073071133 1 1 -1.96550938793341 0.99841576443763]  LatticeCoeffs=[0.2 0.4]  denIgnore=on  FiltPerSampPopup=One filter per frame  IC=0  ICnum=0  ICden=0  roundingMode=Floor  overflowMode=off  ScaleValues=[0.944998002113535;1;1;1;1;1;1;1;1;1;1;1;1;1]  scaleValueFracLength=14  stageInFracLength=15  stageOutFracLength=15  FilterSource=Specify via dialog  dfiltObjectName=dfilt.dffir([1 2 1])
  Stage5 : dsparch4/Digital Filter  Tag=BlockMethodSubSystem  DialogController=dspdialog.DigitalFilter  DialogControllerArgs=DataTag26  TypePopup=IIR (poles & zeros)  IIRFiltStruct=Biquad direct form II (SOS)  AllPoleFiltStruct=Direct form  FIRFiltStruct=Direct form  CoeffSource=Specify via dialog  NumCoeffs=[1 2]  DenCoeffs=[1 0.1]  BiQuadCoeffs=[1 -1.94478249891763 1 1 -1.93168563103253 0.986531277515732;1 -1.94478249891763 1 1 -1.93122059433768 0.98683224264617;1 -1.94478249891763 1 1 -1.93289679174763 0.987008022660797;1 -1.94478249891763 1 1 -1.9315440207779 0.987909159177024;1 -1.94478249891763 1 1 -1.93477174408612 0.988220764886103;1 -1.94478249891763 1 1 -1.93265238090657 0.989713390126836;1 -1.94478249891763 1 1 -1.93719562555007 0.990089878461174;1 -1.94478249891763 1 1 -1.93449307371312 0.99214912798033;1 -1.94478249891763 1 1 -1.94002906949208 0.992504525913789;1 -1.94478249891763 1 1 -1.93696481960067 0.995076908665192;1 -1.94478249891763 1 1 -1.94311601779459 0.995329644404817;1 -1.94478249891763 1 1 -1.93992220998769 0.998321181982756;1 -1.94478249891763 1 1 -1.94629090980952 0.998412672723036]  LatticeCoeffs=[0.2 0.4]  denIgnore=on  FiltPerSampPopup=One filter per frame  IC=0  ICnum=0  ICden=0  roundingMode=Floor  overflowMode=off  ScaleValues=[0.945304374468395;1;1;1;1;1;1;1;1;1;1;1;1;1]  scaleValueFracLength=14  stageInFracLength=15  stageOutFracLength=15  FilterSource=Specify via dialog  dfiltObjectName=dfilt.dffir([1 2 1])
  Stage6 : dsparch4/Digital Filter  Tag=BlockMethodSubSystem  DialogController=dspdialog.DigitalFilter  DialogControllerArgs=DataTag27  TypePopup=IIR (poles & zeros)  IIRFiltStruct=Biquad direct form II (SOS)  AllPoleFiltStruct=Direct form  FIRFiltStruct=Direct form  CoeffSource=Specify via dialog  NumCoeffs=[1 2]  DenCoeffs=[1 0.1]  BiQuadCoeffs=[1 -1.92064508859285 1 1 -1.90765410756011 0.986472273185828;1 -1.92064508859285 1 1 -1.907050442905 0.986789562567385;1 -1.92064508859285 1 1 -1.90899779890478 0.986936076758397;1 -1.92064508859285 1 1 -1.90723446074659 0.987882764412469;1 -1.92064508859285 1 1 -1.91099420923453 0.988142502047033;1 -1.92064508859285 1 1 -1.90820859710794 0.989700395733405;1 -1.92064508859285 1 1 -1.91352351788692 0.990014235945716;1 -1.92064508859285 1 1 -1.90992699967146 0.992144970754847;1 -1.92064508859285 1 1 -1.91644123248104 0.992441250621335;1 -1.92064508859285 1 1 -1.91229576801519 0.995076816055327;1 -1.92064508859285 1 1 -1.91958607166706 0.995287523829068;1 -1.92064508859285 1 1 -1.91517702031526 0.998321590786422;1 -1.92064508859285 1 1 -1.92278752399999 0.998397870496279]  LatticeCoeffs=[0.2 0.4]  denIgnore=on  FiltPerSampPopup=One filter per frame  IC=0  ICnum=0  ICden=0  roundingMode=Floor  overflowMode=off  ScaleValues=[0.94506988263773;1;1;1;1;1;1;1;1;1;1;1;1;1]  scaleValueFracLength=14  stageInFracLength=15  stageOutFracLength=15  FilterSource=Specify via dialog  dfiltObjectName=dfilt.dffir([1 2 1])
  Stage7 : dsparch4/Digital Filter  Tag=BlockMethodSubSystem  DialogController=dspdialog.DigitalFilter  DialogControllerArgs=DataTag28  TypePopup=IIR (poles & zeros)  IIRFiltStruct=Biquad direct form II (SOS)  AllPoleFiltStruct=Direct form  FIRFiltStruct=Direct form  CoeffSource=Specify via dialog  NumCoeffs=[1 2]  DenCoeffs=[1 0.1]  BiQuadCoeffs=[1 -1.89222757165677 1 1 -1.87946492530582 0.986510453032056;1 -1.89222757165677 1 1 -1.87872413047093 0.986838101460465;1 -1.89222757165677 1 1 -1.88093278114135 0.986961705641337;1 -1.89222757165677 1 1 -1.87876382191273 0.987936924736541;1 -1.89222757165677 1 1 -1.88303530627035 0.988156052672692;1 -1.89222757165677 1 1 -1.87959304768991 0.989753596101735;1 -1.89222757165677 1 1 -1.88564809933575 0.990018375641976;1 -1.89222757165677 1 1 -1.88117342448449 0.992189935251698;1 -1.89222757165677 1 1 -1.88862249944903 0.992439907123505;1 -1.89222757165677 1 1 -1.88341916121208 0.995106934972423;1 -1.89222757165677 1 1 -1.89179355317212 0.99528471353657;1 -1.89222757165677 1 1 -1.88620064251826 0.998332207367685;1 -1.89222757165677 1 1 -1.89498786374351 0.998396566697007]  LatticeCoeffs=[0.2 0.4]  denIgnore=on  FiltPerSampPopup=One filter per frame  IC=0  ICnum=0  ICden=0  roundingMode=Floor  overflowMode=off  ScaleValues=[0.945221609871693;1;1;1;1;1;1;1;1;1;1;1;1;1]  scaleValueFracLength=14  stageInFracLength=15  stageOutFracLength=15  FilterSource=Specify via dialog  dfiltObjectName=dfilt.dffir([1 2 1])
  Stage8 : dsparch4/Digital Filter  Tag=BlockMethodSubSystem  DialogController=dspdialog.DigitalFilter  DialogControllerArgs=DataTag29  TypePopup=IIR (poles & zeros)  IIRFiltStruct=Biquad direct form II (SOS)  AllPoleFiltStruct=Direct form  FIRFiltStruct=Direct form  CoeffSource=Specify via dialog  NumCoeffs=[1 2]  DenCoeffs=[1 0.1]  BiQuadCoeffs=[1 -1.85960883542276 1 1 -1.84593411646957 0.986021509148453;1 -1.85960883542276 1 1 -1.84734605082752 0.986086207824345;1 -1.85960883542276 1 1 -1.84544140778377 0.986909714475135;1 -1.85960883542276 1 1 -1.84957097535378 0.987086633043367;1 -1.85960883542276 1 1 -1.84591485590852 0.9887038952601;1 -1.85960883542276 1 1 -1.85245319647007 0.988945992272582;1 -1.85960883542276 1 1 -1.8473354240394 0.991292677324705;1 -1.85960883542276 1 1 -1.85579926237776 0.991535378665241;1 -1.85960883542276 1 1 -1.84961594661188 0.994504963105796;1 -1.85960883542276 1 1 -1.85939042619789 0.994683183912115;1 -1.85960883542276 1 1 -1.85260449337881 0.998120129074157;1 -1.85960883542276 1 1 -1.86299517573272 0.998185591844758]  LatticeCoeffs=[0.2 0.4]  denIgnore=on  FiltPerSampPopup=One filter per frame  IC=0  ICnum=0  ICden=0  roundingMode=Floor  overflowMode=off  ScaleValues=[0.947184039013874;1;1;1;1;1;1;1;1;1;1;1;1]  scaleValueFracLength=14  stageInFracLength=15  stageOutFracLength=15  FilterSource=Specify via dialog  dfiltObjectName=dfilt.dffir([1 2 1])
  Stage9 : dsparch4/Digital Filter  Tag=BlockMethodSubSystem  DialogController=dspdialog.DigitalFilter  DialogControllerArgs=DataTag30  TypePopup=IIR (poles & zeros)  IIRFiltStruct=Biquad direct form II (SOS)  AllPoleFiltStruct=Direct form  FIRFiltStruct=Direct form  CoeffSource=Specify via dialog  NumCoeffs=[1 2]  DenCoeffs=[1 0.1]  BiQuadCoeffs=[1 -1.82286130163383 1 1 -1.8093904390343 0.986049340185928;1 -1.82286130163383 1 1 -1.81095051165661 0.986105875757923;1 -1.82286130163383 1 1 -1.80873514996766 0.986943025633069;1 -1.82286130163383 1 1 -1.81330095324135 0.987097623443224;1 -1.82286130163383 1 1 -1.80904088159003 0.988738220453347;1 -1.82286130163383 1 1 -1.81627907594021 0.988949776437469;1 -1.82286130163383 1 1 -1.81029885913928 0.991322642616634;1 -1.82286130163383 1 1 -1.81968568641089 0.991534729877009;1 -1.82286130163383 1 1 -1.81243274513281 0.994525446348993;1 -1.82286130163383 1 1 -1.82329772701486 0.994681188352925;1 -1.82286130163383 1 1 -1.8153013406224 0.998127421634027;1 -1.82286130163383 1 1 -1.82688113842232 0.998184627861444]  LatticeCoeffs=[0.2 0.4]  denIgnore=on  FiltPerSampPopup=One filter per frame  IC=0  ICnum=0  ICden=0  roundingMode=Floor  overflowMode=off  ScaleValues=[0.947272180688283;1;1;1;1;1;1;1;1;1;1;1;1]  scaleValueFracLength=14  stageInFracLength=15  stageOutFracLength=15  FilterSource=Specify via dialog  dfiltObjectName=dfilt.dffir([1 2 1])
  Out : Outport
  wires:
  In/1 -> Stage1/1
  Stage1/1 -> Stage2/1
  Stage2/1 -> Stage3/1
  Stage3/1 -> Stage4/1
  Stage4/1 -> Stage5/1
  Stage5/1 -> Stage6/1
  Stage6/1 -> Stage7/1
  Stage7/1 -> Stage8/1
  Stage8/1 -> Stage9/1
  Stage9/1 -> Stage10/1
  Stage10/1 -> Out/1
